simulink model "simulink_ReachCG"  (R2021a)
settings: Solver=ode45  StartTime=0.0  StopTime=130*Ts  RelTol=1e-3  EnableMultiTasking=on
undefined symbols (not defined in the file or in its folder): DiscIntNeverNeededParam
settings Model: Creator=MatFlo  LastModifiedBy=Mannaiyar
settings SolverCC: AlgebraicLoopSolver=TrustRegion
settings DataIOCC: LimitDataPoints=on  SaveFormat=Array  SignalLoggingSaveFormat=ModelDataLogs  ReturnWorkspaceOutputs=off
settings OptimizationCC: ExpressionDepthLimit=2147483647  LifeSpan=inf
settings DebuggingCC: UnderspecifiedInitializationDetection=Classic  MergeDetectMultiDrivingBlocksExec=none  SolverPrmCheckMsg=warning  FcnCallInpInsideContextMsg=warning  StateNameClashWarn=warning  SFUnexpectedBacktrackingDiag=warning  SFNoUnconditionalDefaultTransitionDiag=warning  SFExecutionAtInitializationDiag=none  SFMachineParentedDataDiag=warning  ArithmeticOperatorsInVariantConditions=warning
settings HardwareCC: ProdBitPerPointer=32  ProdBitPerSizeT=32  ProdBitPerPtrDiffT=32  ProdLargestAtomicFloat=None  ProdIntDivRoundTo=Undefined  ProdEndianess=Unspecified  ProdWordSize=32  ProdHWDeviceType=32-bit Generic
settings ModelReferenceCC: PropagateSignalLabelsOutOfModel=off
settings SFSimCC: SimUseLocalCustomCode=off  CustomCodeUndefinedFunction=UseInterfaceOnly
settings RTWCC: RTWUseLocalCustomCode=off
settings CodeAppCC: StateflowObjectComments=on
settings GRTTargetCC: TargetLangStandard=C89/C90 (ANSI)  CombineOutputUpdateFcns=off  GRTInterface=on
settings ConfigComp: CovMetricSettings=dw  CovSaveCumulativeToWorkspaceVar=on  CovSaveSingleToWorkspaceVar=on  CovExternalEMLEnable=off

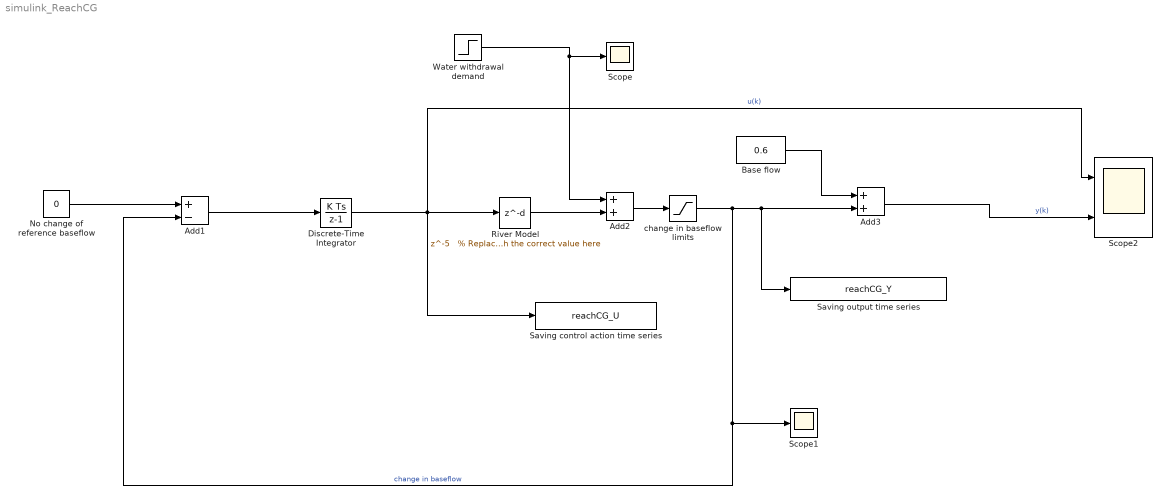
== system simulink_ReachCG ==
  " Water withdrawal demand " : Step  Time="105    % Replace 0 with the correct value here"  Before="0   % Replace 0 with the correct value here"  After="-0.4    % Replace 0 with the correct value here"  SampleTime="5   % hours"
  Add1 : Sum  Inputs=+-  SampleTime=5
  Add2 : Sum  SampleTime=5
  Add3 : Sum  SampleTime=5
  Base flow : Constant  Value=0.6  SampleTime=-1
  Discrete-Time Integrator : DiscreteIntegrator  gainval="0.01       % Replace 1 with the correct value here"  SampleTime="5     % hours"  ICPrevOutput=DiscIntNeverNeededParam  ICPrevScaledInput=DiscIntNeverNeededParam
  No change of reference baseflow : Constant  Value=0
  River Model : Delay  DelayLength="5   % Replace 1 with the correct value here"  SampleTime="5    % hours"
  Saving control action time series : ToFile  Filename=reachCG_U  MatrixName=rU  SampleTime=5
  Saving output time series : ToFile  Filename=reachCG_Y  MatrixName=rY  SampleTime=5
  Scope : Scope
  Scope1 : Scope
  Scope2 : Scope  NumInputPorts=2
  change in baseflow limits : Saturate  UpperLimit=0.3  LowerLimit=-0.3  SampleTime="5    % hours"
  wires:
  No change of reference baseflow/1 -> Add1/1
  Add1/1 -> Discrete-Time Integrator/1
  River Model/1 -> Add2/2
  Add3/1 -> Scope2/2  "y(k)"
  Base flow/1 -> Add3/1
  " Water withdrawal demand "/1 -> Add2/1, Scope/1
  Discrete-Time Integrator/1 -> Scope2/1, River Model/1, Saving control action time series/1  "u(k)"
  Add2/1 -> change in baseflow limits/1
  change in baseflow limits/1 -> Add3/2, Saving output time series/1, Scope1/1, Add1/2  "change in baseflow"
